simulink model "SingleVehicle_HIL"  (R2016b)
settings: Solver=ode4  StartTime=0.0  StopTime=inf  FixedStep=0.01  RelTol=1e-3  EnableMultiTasking=on
undefined symbols (not defined in the file or in its folder): Angular, dpsi, FromPrescan, IdealSensors, Linear, psi, RHSC, RHSCCmdBus, v, wpFollower, y
undefined symbols (not defined in the file): vd
libraries: robotlib x6, sldrtlib x1
(part 1 of 2)
Description:
  | Real-Time Van der Pol Simulation
  | 
  | The example model "sldrtex_vdp" shows a real-time version of the Simulink(R) Van der Pol
  | simulation model. This model does not need any external signals, so it does
  | not need any data acquisition hardware or driver. This makes the model ideal
  | for the first experiments with Simulink Desktop Real-Time(TM), without need to
  | worry about proper I/O hardware configuration.
  | 
  | How to run this model in Normal Mode:
  | 
  | 1) Double-click the orange button to switch to Normal Mode if needed.
  | 2) Start the real-time execution using Simulation->Run.
  | 3) Observe any missed ticks on the Missed Ticks scope.
  | 
  | How to run this model in External Mode:
  | 
  | 1) Double-click the orange button to switch to External Mode if needed.
  | 2) Start the real-time execution using Simulation->Run. The model will automatically
  |    build, connect to Simulink in External Mode and start.
  | 3) Missed ticks will be always zero.
settings Model: ExtModeTrigDuration=101  Creator=The MathWorks, Inc.  LastModifiedBy=yutongli
settings DataIOCC: LimitDataPoints=on  SignalLoggingName=logsOut
settings OptimizationCC: ExpressionDepthLimit=2147483647  InitFltsAndDblsToZero=on  EfficientMapNaN2IntZero=off  LifeSpan=inf
settings DebuggingCC: UnderspecifiedInitializationDetection=Classic  MergeDetectMultiDrivingBlocksExec=none  SignalResolutionControl=TryResolveAllWithWarning  FcnCallInpInsideContextMsg=warning  AllowSymbolicDim=off  StateNameClashWarn=warning  SFUnexpectedBacktrackingDiag=warning  SFNoUnconditionalDefaultTransitionDiag=warning  SFExecutionAtInitializationDiag=none
settings HardwareCC: TargetBitPerLong=64  TargetBitPerPointer=64  TargetBitPerSizeT=64  TargetBitPerPtrDiffT=64  TargetIntDivRoundTo=Zero  TargetEndianess=LittleEndian  TargetWordSize=64  TargetHWDeviceType=Intel->x86-64
settings ModelReferenceCC: PropagateSignalLabelsOutOfModel=off
settings RTWCC: SystemTargetFile=sldrt.tlc  TemplateMakefile=sldrt.tmf  Description=Simulink Desktop Real-Time  RTWCompilerOptimization=on
settings CodeAppCC: MaxIdLength=95
settings SimulinkDesktopRealTimeCC: TargetPreCompLibLocation=C:\Program Files\MATLAB\R2016B\toolbox\sldrt\lib\win64  TargetLangStandard=C89/C90 (ANSI)  GeneratePreprocessorConditionals=Disable all  SupportVariableSizeSignals=off
settings ConfigComp: CovMetricSettings=dw  CovHtmlReporting=on  CovSaveCumulativeToWorkspaceVar=on  CovSaveSingleToWorkspaceVar=on  CovShowResultsExplorer=off  CovExternalEMLEnable=off  CovSFcnEnable=off

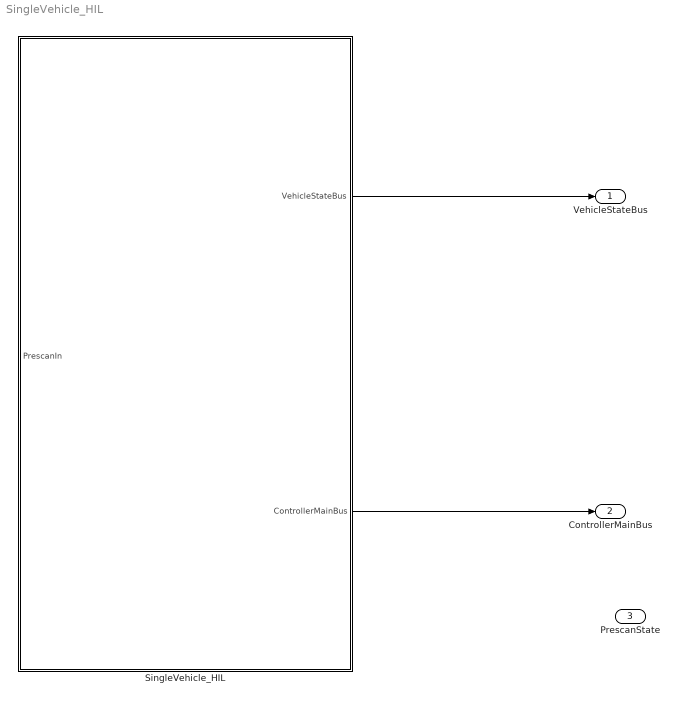
== system SingleVehicle_HIL ==
  SingleVehicle_HIL : Subsystem  mask{veh_struct=vd}
      mask prompts: veh_struct "Vehicle Parameter Structure"
      mask init:
      | set_param([gcb,'/Monitor/VehicleStateBusStorage'],'VariableName',[get_param(gcb,'MaskValueString'),'_DataVehicleBus']);
      | set_param([gcb,'/Monitor/ControllerMainBusStorage/ArbitratedActuationReqStorage'],'VariableName', ...
      |     [get_param(gcb,'MaskValueString'),'_DataControllerMain_ArbitrationActuationReq']);
      | set_param([gcb,'/Monitor/ControllerMainBusStorage/wpFollowerStorage'],'VariableName', ...
      |     [get_param(gcb,'MaskValueString'),'_DataControllerMain_wpFollower']);
      | set_param([gcb,'/Monitor/ControllerMainBusStorage/finalWayPointStorarge'],'VariableName', ...
      |     [get_param(gcb,'MaskValueString'),'_DataControllerMain_finalWayPoint']);
      | set_param([gcb,'/Monitor/ControllerMainBusStorage/currentWayPointStorage'],'VariableName', ...
      |     [get_param(gcb,'MaskValueString'),'_DataControllerMain_currentWayPoint']);
      | set_param([gcb,'/Monitor/ControllerMainBusStorage/wayPointArrayStorage'],'VariableName', ...
      |     [get_param(gcb,'MaskValueString'),'_DataControllerMain_wayPointArray']);
      | set_param([gcb,'/Monitor/ControllerMainBusStorage/selfAwareessBusStorage'],'VariableName', ...
      |     [get_param(gcb,'MaskValueString'),'_DataControllerMain_selfAwareessBus']);
      | set_param([gcb,'/Monitor/ControllerMainBusStorage/IdealSensorsStorage'],'VariableName', ...
      |     [get_param(gcb,'MaskValueString'),'_DataControllerMain_IdealSensors']);
      | set_param([gcb,'/Monitor/ControllerMainBusStorage/FromPrescanStorage'],'VariableName', ...
      |     [get_param(gcb,'MaskValueString'),'_DataControllerMain_FromPrescan']);
  VehicleStateBus : Outport
  ControllerMainBus : Outport  Port=2
  PrescanState : Outport  Port=3
  wires:
  SingleVehicle_HIL/1(VehicleStateBus) -> VehicleStateBus/1
  SingleVehicle_HIL/2(ControllerMainBus) -> ControllerMainBus/1
  ? -> PrescanState/1

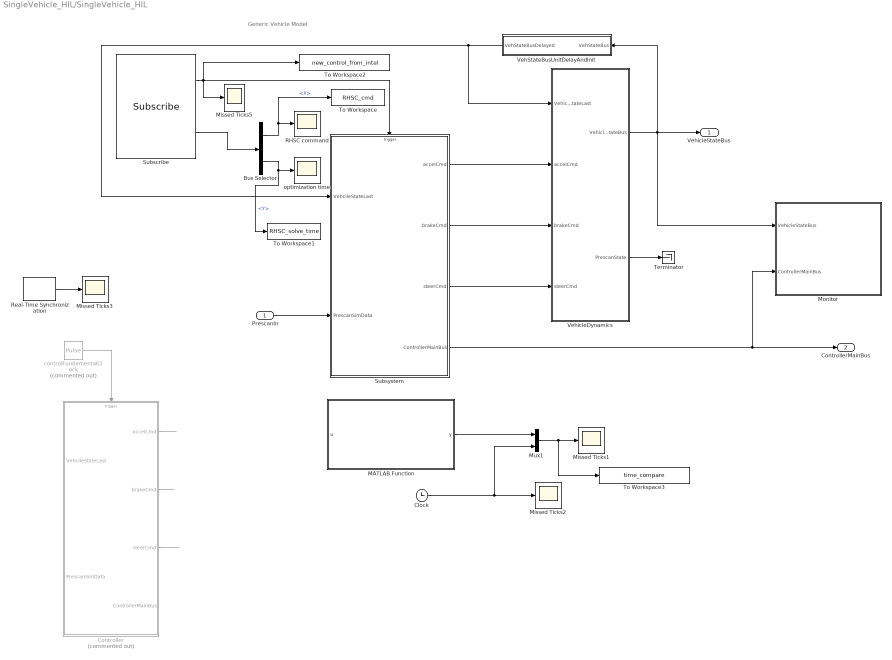
== system SingleVehicle_HIL/SingleVehicle_HIL ==
  note: Generic Vehicle Model
  PrescanIn : Inport
  Bus Selector : BusSelector  OutputSignals=Linear.X,Linear.Y
  Clock : Clock
  Controller : Subsystem  Commented=on
  MATLAB Function : MATLAB Function  TreatAsAtomicUnit=on
  Missed Ticks{1..3,5} (4 alike) : Scope
  Monitor : Subsystem
  Mux1 : Mux  Inputs=2
  RHSC command : Scope
  Real-Time Synchronization : sldrtlib/Real-Time Synchronization  SampleTime=0.01  MaxMissedTicks=1000  ShowMissedTicks=on  YieldWhenWaiting=off
  Subscribe : robotlib/Subscribe  SourceLibraryInfo=This block requires Robotics System Toolbox  topicSource=Select from ROS network  topic=/RHSC_cmd  messageType=geometry_msgs/Twist  sampleTime=-1  messageQueueLength=1
  Subsystem : Subsystem
  Terminator : Terminator
  To Workspace : ToWorkspace  VariableName=RHSC_cmd  SaveFormat=Structure With Time  SampleTime=-1
  To Workspace1 : ToWorkspace  VariableName=RHSC_solve_time  SaveFormat=Structure With Time  SampleTime=-1
  To Workspace2 : ToWorkspace  VariableName=new_control_from_intel  SaveFormat=Structure With Time  SampleTime=-1
  To Workspace3 : ToWorkspace  VariableName=time_compare  SaveFormat=Structure With Time  SampleTime=-1
  VehStateBusUnitDelayAndInit : Subsystem
  VehicleDynamics : Subsystem
  controlFundamentalClock : DiscretePulseGenerator  Commented=on  PulseType=Time based  Period=veh_struct.CONTROL_OS_SAMPLETIME  PulseWidth=5
  optimization time : Scope
  VehicleStateBus : Outport
  ControllerMainBus : Outport  Port=2
  wires:
  PrescanIn/1 -> Subsystem/2(PrescanSimData)
  Controller/1(accelCmd) -> ?
  Controller/2(brakeCmd) -> ?
  Controller/3(steerCmd) -> ?
  VehicleDynamics/1(VehicleStateBus) -> VehStateBusUnitDelayAndInit/1(VehStateBus), Monitor/1(VehicleStateBus), VehicleStateBus/1
  VehStateBusUnitDelayAndInit/1(VehStateBusDelayed) -> Subsystem/1(VehcileStateLast), VehicleDynamics/1(VehicleStateLast)
  controlFundamentalClock/1 -> Controller/Trigger
  Real-Time Synchronization/1 -> Missed Ticks3/1
  MATLAB Function/1(y) -> Mux1/1
  Mux1/1 -> To Workspace3/1, Missed Ticks1/1
  Clock/1 -> Missed Ticks2/1, Mux1/2
  Subscribe/1 -> To Workspace2/1, Subsystem/Trigger, Missed Ticks5/1
  Subscribe/2 -> Bus Selector/1
  Bus Selector/1 -> RHSC command/1, To Workspace/1  "<X>"
  Subsystem/4(ControllerMainBus) -> Monitor/2(ControllerMainBus), ControllerMainBus/1
  Subsystem/1(accelCmd) -> VehicleDynamics/2(accelCmd)
  Subsystem/2(brakeCmd) -> VehicleDynamics/3(brakeCmd)
  Subsystem/3(steerCmd) -> VehicleDynamics/4(steerCmd)
  VehicleDynamics/2(PrescanState) -> Terminator/1
  Bus Selector/2 -> To Workspace1/1, optimization time/1  "<Y>"

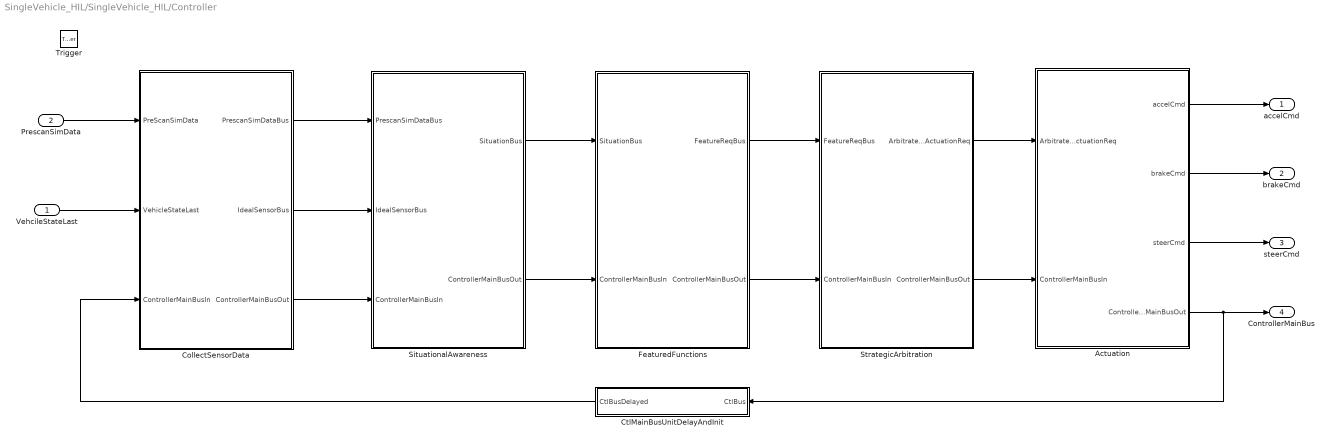
== system SingleVehicle_HIL/SingleVehicle_HIL/Controller ==
  VehcileStateLast : Inport
  PrescanSimData : Inport  Port=2
  Trigger : TriggerPort  VariantControl=Variant  PortDimensions=1
  Actuation : Subsystem
  CollectSensorData : Subsystem
  CtlMainBusUnitDelayAndInit : Subsystem
  FeaturedFunctions : Subsystem
  SituationalAwareness : Subsystem
  StrategicArbitration : Subsystem
  accelCmd : Outport
  brakeCmd : Outport  Port=2
  steerCmd : Outport  Port=3
  ControllerMainBus : Outport  Port=4
  wires:
  PrescanSimData/1 -> CollectSensorData/1(PreScanSimData)
  Actuation/1(accelCmd) -> accelCmd/1
  Actuation/2(brakeCmd) -> brakeCmd/1
  Actuation/3(steerCmd) -> steerCmd/1
  StrategicArbitration/1(ArbitratedActuationReq) -> Actuation/1(ArbitratedActuationReq)
  StrategicArbitration/2(ControllerMainBusOut) -> Actuation/2(ControllerMainBusIn)
  FeaturedFunctions/2(ControllerMainBusOut) -> StrategicArbitration/2(ControllerMainBusIn)
  FeaturedFunctions/1(FeatureReqBus) -> StrategicArbitration/1(FeatureReqBus)
  SituationalAwareness/1(SituationBus) -> FeaturedFunctions/1(SituationBus)
  SituationalAwareness/2(ControllerMainBusOut) -> FeaturedFunctions/2(ControllerMainBusIn)
  CollectSensorData/3(ControllerMainBusOut) -> SituationalAwareness/3(ControllerMainBusIn)
  VehcileStateLast/1 -> CollectSensorData/2(VehicleStateLast)
  Actuation/4(ControllerMainBusOut) -> CtlMainBusUnitDelayAndInit/1(CtlBus), ControllerMainBus/1
  CtlMainBusUnitDelayAndInit/1(CtlBusDelayed) -> CollectSensorData/3(ControllerMainBusIn)
  CollectSensorData/1(PrescanSimDataBus) -> SituationalAwareness/1(PrescanSimDataBus)
  CollectSensorData/2(IdealSensorBus) -> SituationalAwareness/2(IdealSensorBus)

== system SingleVehicle_HIL/SingleVehicle_HIL/Monitor ==
  VehicleStateBus : Inport
  ControllerMainBus : Inport  Port=2
  ControllerMainBusStorage : Subsystem
  VehicleStateBusStorage : ToWorkspace  VariableName=vd_DataVehicleBus  SaveFormat=Timeseries  SampleTime=-1
  wires:
  VehicleStateBus/1 -> VehicleStateBusStorage/1
  ControllerMainBus/1 -> ControllerMainBusStorage/1(ControllerMainBus)

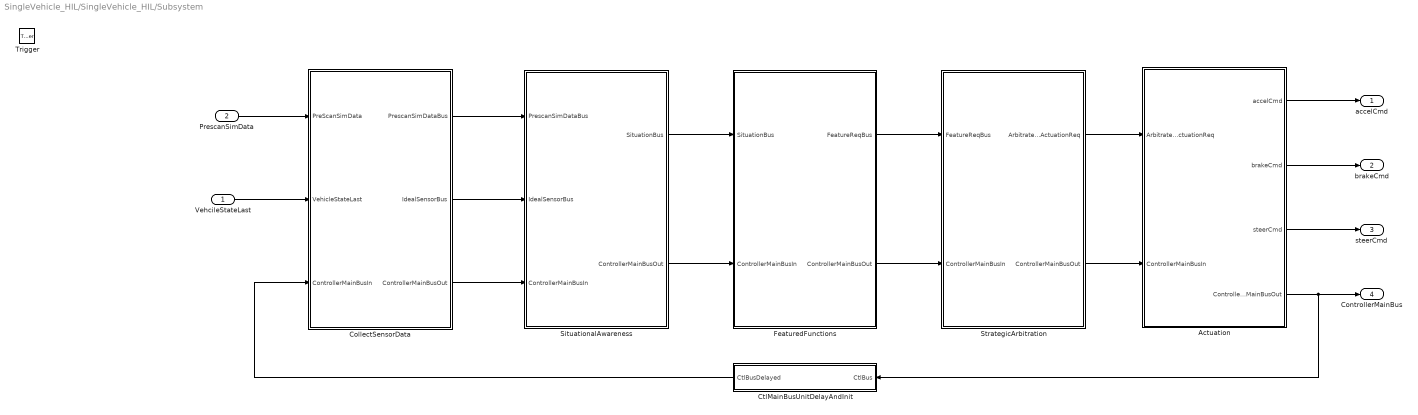
== system SingleVehicle_HIL/SingleVehicle_HIL/Subsystem ==
  VehcileStateLast : Inport
  PrescanSimData : Inport  Port=2
  Trigger : TriggerPort  VariantControl=Variant  PortDimensions=1
  Actuation : Subsystem
  CollectSensorData : Subsystem
  CtlMainBusUnitDelayAndInit : Subsystem
  FeaturedFunctions : Subsystem
  SituationalAwareness : Subsystem
  StrategicArbitration : Subsystem
  accelCmd : Outport
  brakeCmd : Outport  Port=2
  steerCmd : Outport  Port=3
  ControllerMainBus : Outport  Port=4
  wires:
  PrescanSimData/1 -> CollectSensorData/1(PreScanSimData)
  Actuation/1(accelCmd) -> accelCmd/1
  Actuation/2(brakeCmd) -> brakeCmd/1
  Actuation/3(steerCmd) -> steerCmd/1
  StrategicArbitration/1(ArbitratedActuationReq) -> Actuation/1(ArbitratedActuationReq)
  StrategicArbitration/2(ControllerMainBusOut) -> Actuation/2(ControllerMainBusIn)
  FeaturedFunctions/2(ControllerMainBusOut) -> StrategicArbitration/2(ControllerMainBusIn)
  FeaturedFunctions/1(FeatureReqBus) -> StrategicArbitration/1(FeatureReqBus)
  SituationalAwareness/1(SituationBus) -> FeaturedFunctions/1(SituationBus)
  SituationalAwareness/2(ControllerMainBusOut) -> FeaturedFunctions/2(ControllerMainBusIn)
  CollectSensorData/3(ControllerMainBusOut) -> SituationalAwareness/3(ControllerMainBusIn)
  VehcileStateLast/1 -> CollectSensorData/2(VehicleStateLast)
  Actuation/4(ControllerMainBusOut) -> CtlMainBusUnitDelayAndInit/1(CtlBus), ControllerMainBus/1
  CtlMainBusUnitDelayAndInit/1(CtlBusDelayed) -> CollectSensorData/3(ControllerMainBusIn)
  CollectSensorData/1(PrescanSimDataBus) -> SituationalAwareness/1(PrescanSimDataBus)
  CollectSensorData/2(IdealSensorBus) -> SituationalAwareness/2(IdealSensorBus)

== system SingleVehicle_HIL/SingleVehicle_HIL/VehStateBusUnitDelayAndInit ==
  VehStateBus : Inport
  MATLAB Function : MATLAB Function  TreatAsAtomicUnit=on
  Memory : Memory  InheritSampleTime=on
  VehStateBusDelayed : Outport
  wires:
  Memory/1 -> MATLAB Function/1(u)
  VehStateBus/1 -> Memory/1
  MATLAB Function/1(y) -> VehStateBusDelayed/1

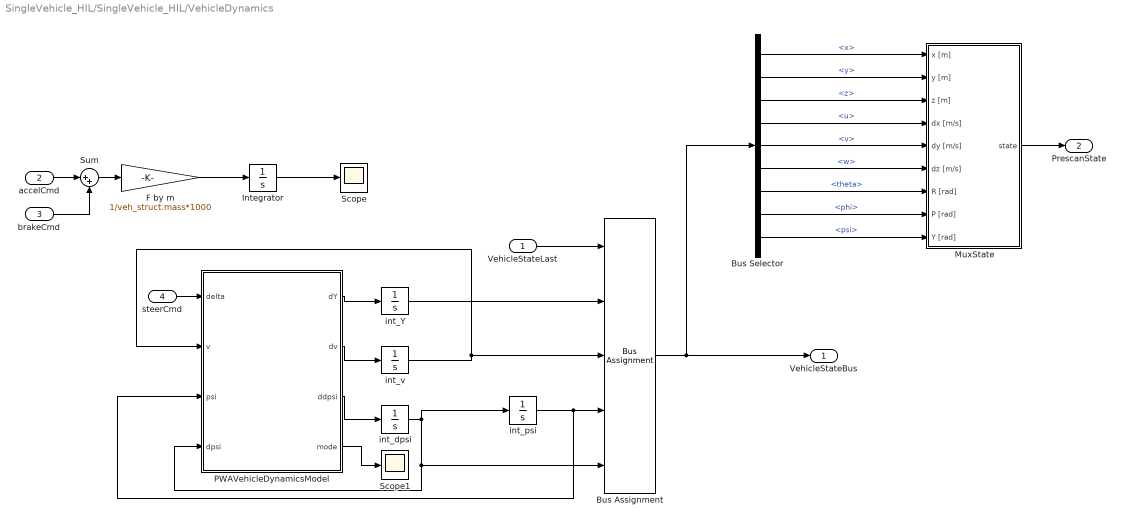
== system SingleVehicle_HIL/SingleVehicle_HIL/VehicleDynamics ==
  VehicleStateLast : Inport
  accelCmd : Inport  Port=2
  brakeCmd : Inport  Port=3
  steerCmd : Inport  Port=4
  Bus Assignment : BusAssignment  AssignedSignals=y,v,psi,dpsi
  Bus Selector : BusSelector  OutputSignals=x,y,z,u,v,w,theta,phi,psi
  F by m : Gain  Gain=1/veh_struct.mass*1000
  Integrator : Integrator  InitialCondition=veh_struct.init.u
  MuxState : Subsystem  Tag=MuxState  mask(Empty Dynamics State Block){positioningmode=on, TimeStep=1/20}
      mask prompts: positioningmode "Positioning Mode"; TimeStep "Auto Assigned: Time Step [s]"
      mask help:
      | Build the state of an actor based on user input.
      | The user can either use positioning mode or dynamics mode.
      | - When using positioning mode the position and orientation of the actor are set directly based on the input. Expected input is relative to the initial position and orientation of the actor. It's also possible to specify the velocity of the actor, though this input isn't used, only passed on.
      | - When using dynamics mode the position input is ignored. Expected input is velocity and orientation. The velocity is relative the current orientation of the actor, while orientation is relative to its initial orientation. The position of the actor is calculated based on the velocity and orientation given.
      settings: DeleteFcn=PreScanBlockDeleteFcn;
  PWAVehicleDynamicsModel : MATLAB Function  TreatAsAtomicUnit=on
  Scope : Scope
  Scope1 : Scope
  Sum : Sum  Inputs=|++
  int_Y : Integrator  InitialCondition=veh_struct.init.Y
  int_dpsi : Integrator  InitialCondition=veh_struct.init.dpsi
  int_psi : Integrator  InitialCondition=veh_struct.init.psi
  int_v : Integrator  InitialCondition=veh_struct.init.v
  VehicleStateBus : Outport
  PrescanState : Outport  Port=2
  wires:
  MuxState/1(state) -> PrescanState/1
  Bus Assignment/1 -> VehicleStateBus/1, Bus Selector/1
  Bus Selector/3 -> MuxState/3(z [m])  "<z>"
  Bus Selector/4 -> MuxState/4(dx [m/s])  "<u>"
  Bus Selector/5 -> MuxState/5(dy [m/s])  "<v>"
  Bus Selector/6 -> MuxState/6(dz [m/s])  "<w>"
  Bus Selector/1 -> MuxState/1(x [m])  "<x>"
  Bus Selector/2 -> MuxState/2(y [m])  "<y>"
  Bus Selector/7 -> MuxState/7(R [rad])  "<theta>"
  Bus Selector/9 -> MuxState/9(Y [rad])  "<psi>"
  Bus Selector/8 -> MuxState/8(P [rad])  "<phi>"
  VehicleStateLast/1 -> Bus Assignment/1
  accelCmd/1 -> Sum/1
  brakeCmd/1 -> Sum/2
  Sum/1 -> F by m/1
  F by m/1 -> Integrator/1
  Integrator/1 -> Scope/1
  steerCmd/1 -> PWAVehicleDynamicsModel/1(delta)
  PWAVehicleDynamicsModel/2(dv) -> int_v/1
  int_v/1 -> PWAVehicleDynamicsModel/2(v), Bus Assignment/3
  PWAVehicleDynamicsModel/3(ddpsi) -> int_dpsi/1
  int_dpsi/1 -> int_psi/1, PWAVehicleDynamicsModel/4(dpsi), Bus Assignment/5
  PWAVehicleDynamicsModel/1(dY) -> int_Y/1
  int_Y/1 -> Bus Assignment/2
  int_psi/1 -> PWAVehicleDynamicsModel/3(psi), Bus Assignment/4
  PWAVehicleDynamicsModel/4(mode) -> Scope1/1

== system SingleVehicle_HIL/SingleVehicle_HIL/Controller/Actuation ==
  ArbitratedActuationReq : Inport
  ControllerMainBusIn : Inport  Port=2
  ActuatorDrivers : Subsystem  TreatAsAtomicUnit=on
  Bus Assignment : BusAssignment  AssignedSignals=ActuationCmdBus
  Bus Selector : BusSelector  OutputSignals=ActuationCmdBus
  DynamicControls : Subsystem  TreatAsAtomicUnit=on
  accelCmd : Outport
  brakeCmd : Outport  Port=2
  steerCmd : Outport  Port=3
  ControllerMainBusOut : Outport  Port=4
  wires:
  ControllerMainBusIn/1 -> DynamicControls/2(Ctl), Bus Assignment/1, Bus Selector/1
  ArbitratedActuationReq/1 -> DynamicControls/1(ActReq)
  Bus Selector/1 -> DynamicControls/3(ActCmdsPrev)  "<ActuationCmdBus>"
  DynamicControls/1(ActCmds) -> ActuatorDrivers/1(ActCmds), Bus Assignment/2
  Bus Assignment/1 -> ControllerMainBusOut/1
  ActuatorDrivers/2(decel_cmd) -> brakeCmd/1
  ActuatorDrivers/1(accel_cmd) -> accelCmd/1
  ActuatorDrivers/3(steering_cmd) -> steerCmd/1

== system SingleVehicle_HIL/SingleVehicle_HIL/Controller/CollectSensorData ==
  PreScanSimData : Inport
  VehicleStateLast : Inport  Port=2
  ControllerMainBusIn : Inport  Port=3
  Bus Assignment : BusAssignment  AssignedSignals=FromPrescan,IdealSensors
  IdealSensorsProcess : Subsystem
  PrescanProcess : Subsystem
  PrescanSimDataBus : Outport
  IdealSensorBus : Outport  Port=2
  ControllerMainBusOut : Outport  Port=3
  wires:
  PreScanSimData/1 -> PrescanProcess/1(PrescanSimData)
  PrescanProcess/1(PrescanSimDataBus) -> Bus Assignment/2, PrescanSimDataBus/1
  VehicleStateLast/1 -> IdealSensorsProcess/1(VehicleState)
  IdealSensorsProcess/1(IdealSensorsBus) -> IdealSensorBus/1, Bus Assignment/3
  Bus Assignment/1 -> ControllerMainBusOut/1
  ControllerMainBusIn/1 -> Bus Assignment/1

== system SingleVehicle_HIL/SingleVehicle_HIL/Controller/CtlMainBusUnitDelayAndInit ==
  CtlBus : Inport
  MATLAB Function : Subsystem  TreatAsAtomicUnit=on
  Memory : Memory  InheritSampleTime=on
  CtlBusDelayed : Outport
  wires:
  Memory/1 -> MATLAB Function/1(u)
  CtlBus/1 -> Memory/1
  MATLAB Function/1(y) -> CtlBusDelayed/1

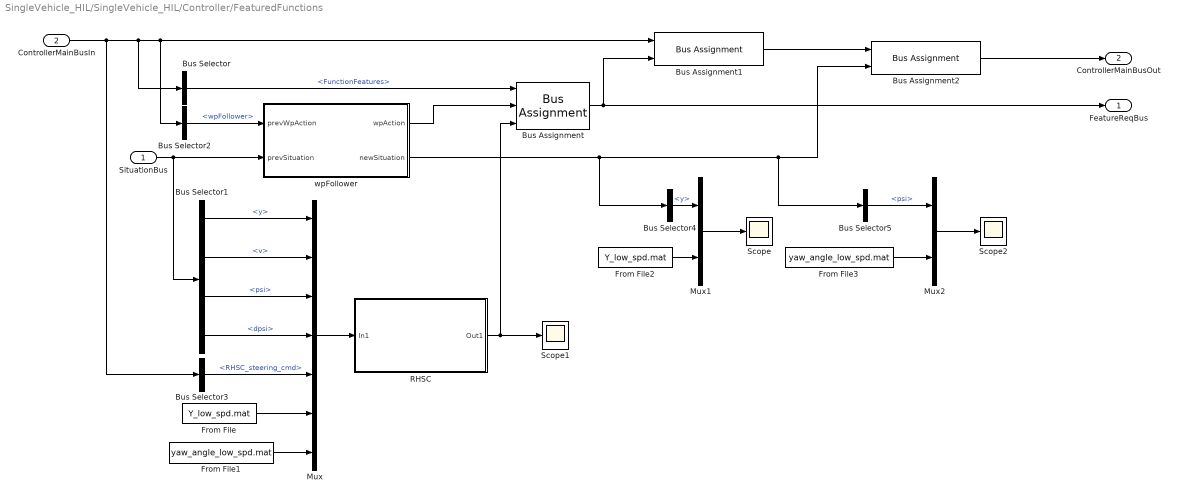
== system SingleVehicle_HIL/SingleVehicle_HIL/Controller/FeaturedFunctions ==
  SituationBus : Inport
  ControllerMainBusIn : Inport  Port=2
  Bus Assignment : BusAssignment  AssignedSignals=wpFollower,RHSCCmdBus.RHSC_steering_cmd
  Bus Assignment1 : BusAssignment  AssignedSignals=FunctionFeatures
  Bus Assignment2 : BusAssignment  AssignedSignals=situationBus
  Bus Selector : BusSelector  OutputSignals=FunctionFeatures
  Bus Selector1 : BusSelector  OutputSignals=selfAwarenessBus.y,selfAwarenessBus.v,selfAwarenessBus.psi,selfAwarenessBus.dpsi
  Bus Selector2 : BusSelector  OutputSignals=FunctionFeatures.wpFollower
  Bus Selector3 : BusSelector  OutputSignals=FunctionFeatures.RHSCCmdBus.RHSC_steering_cmd
  Bus Selector4 : BusSelector  OutputSignals=selfAwarenessBus.y
  Bus Selector5 : BusSelector  OutputSignals=selfAwarenessBus.psi
  From File : FromFile  FileName=Y_low_spd.mat
  From File1 : FromFile  FileName=yaw_angle_low_spd.mat
  From File2 : FromFile  FileName=Y_low_spd.mat
  From File3 : FromFile  FileName=yaw_angle_low_spd.mat
  Mux : Mux  Inputs=7
  Mux1 : Mux  Inputs=2
  Mux2 : Mux  Inputs=2
  RHSC : Subsystem
  Scope : Scope
  Scope1 : Scope
  Scope2 : Scope
  wpFollower : Subsystem  TreatAsAtomicUnit=on
  FeatureReqBus : Outport
  ControllerMainBusOut : Outport  Port=2
  wires:
  ControllerMainBusIn/1 -> Bus Selector3/1, Bus Selector/1, Bus Selector2/1, Bus Assignment1/1
  Bus Selector/1 -> Bus Assignment/1  "<FunctionFeatures>"
  wpFollower/1(wpAction) -> Bus Assignment/2
  Bus Assignment/1 -> Bus Assignment1/2, FeatureReqBus/1
  Bus Assignment1/1 -> Bus Assignment2/1
  wpFollower/2(newSituation) -> Bus Selector4/1, Bus Selector5/1, Bus Assignment2/2
  Bus Assignment2/1 -> ControllerMainBusOut/1
  Bus Selector2/1 -> wpFollower/1(prevWpAction)  "<wpFollower>"
  SituationBus/1 -> Bus Selector1/1, wpFollower/2(prevSituation)
  Bus Selector3/1 -> Mux/5  "<RHSC_steering_cmd>"
  RHSC/1(Out1) -> Scope1/1, Bus Assignment/3
  Mux/1 -> RHSC/1(In1)
  Bus Selector1/1 -> Mux/1  "<y>"
  Bus Selector1/2 -> Mux/2  "<v>"
  Bus Selector1/3 -> Mux/3  "<psi>"
  Bus Selector1/4 -> Mux/4  "<dpsi>"
  From File/1 -> Mux/6
  From File1/1 -> Mux/7
  Bus Selector4/1 -> Mux1/1  "<y>"
  From File2/1 -> Mux1/2
  Mux1/1 -> Scope/1
  Bus Selector5/1 -> Mux2/1  "<psi>"
  From File3/1 -> Mux2/2
  Mux2/1 -> Scope2/1

== system SingleVehicle_HIL/SingleVehicle_HIL/Controller/SituationalAwareness ==
  PrescanSimDataBus : Inport
  IdealSensorBus : Inport  Port=2
  ControllerMainBusIn : Inport  Port=3
  Bus Assignment : BusAssignment  AssignedSignals=situationBus
  Bus Selector : BusSelector  OutputSignals=situationBus
  situationAwareness : Subsystem  TreatAsAtomicUnit=on
  SituationBus : Outport
  ControllerMainBusOut : Outport  Port=2
  wires:
  ControllerMainBusIn/1 -> Bus Assignment/1, Bus Selector/1
  Bus Selector/1 -> situationAwareness/1(prevSituation)  "<situationBus>"
  PrescanSimDataBus/1 -> situationAwareness/2(prescanSimData)
  IdealSensorBus/1 -> situationAwareness/3(idealSensors)
  situationAwareness/1(newSituation) -> Bus Assignment/2, SituationBus/1
  Bus Assignment/1 -> ControllerMainBusOut/1

== system SingleVehicle_HIL/SingleVehicle_HIL/Controller/StrategicArbitration ==
  FeatureReqBus : Inport
  ControllerMainBusIn : Inport  Port=2
  Arbitration : Subsystem  TreatAsAtomicUnit=on
  Bus Assignment : BusAssignment  AssignedSignals=ArbitratedActuationReq
  ArbitratedActuationReq : Outport
  ControllerMainBusOut : Outport  Port=2
  wires:
  FeatureReqBus/1 -> Arbitration/1(FunctionFeatures)
  Arbitration/1(ArbitratedReq) -> Bus Assignment/2, ArbitratedActuationReq/1
  ControllerMainBusIn/1 -> Bus Assignment/1
  Bus Assignment/1 -> ControllerMainBusOut/1

== system SingleVehicle_HIL/SingleVehicle_HIL/Monitor/ControllerMainBusStorage ==
  ControllerMainBus : Inport
  ArbitratedActuationReqStorage : ToWorkspace  VariableName=vd_DataControllerMain_ArbitrationActuationReq  SaveFormat=Timeseries  SampleTime=-1
  Bus Selector : BusSelector  OutputSignals=ArbitratedActuationReq,FunctionFeatures.wpFollower,situationBus.wP.finalWayPoint,situationBus.wP.currentWayPoint,situationBus.wP.wayPointArray,situationBus.selfAwarenessBus,IdealSensors,FromPrescan
  FromPrescanStorage : ToWorkspace  VariableName=vd_DataControllerMain_FromPrescan  SaveFormat=Timeseries  SampleTime=-1
  IdealSensorsStorage : ToWorkspace  VariableName=vd_DataControllerMain_IdealSensors  SaveFormat=Timeseries  SampleTime=-1
  currentWayPointStorage : ToWorkspace  VariableName=vd_DataControllerMain_currentWayPoint  SaveFormat=Timeseries  SampleTime=-1
  finalWayPointStorarge : ToWorkspace  VariableName=vd_DataControllerMain_finalWayPoint  SaveFormat=Timeseries  SampleTime=-1
  selfAwareessBusStorage : ToWorkspace  VariableName=vd_DataControllerMain_selfAwareessBus  SaveFormat=Timeseries  SampleTime=-1
  wayPointArrayStorage : ToWorkspace  VariableName=vd_DataControllerMain_wayPointArray  SampleTime=-1
  wpFollowerStorage : ToWorkspace  VariableName=vd_DataControllerMain_wpFollower  SaveFormat=Timeseries  SampleTime=-1
  wires:
  ControllerMainBus/1 -> Bus Selector/1
  Bus Selector/1 -> ArbitratedActuationReqStorage/1  "<ArbitratedActuationReq>"
  Bus Selector/2 -> wpFollowerStorage/1  "<wpFollower>"
  Bus Selector/3 -> finalWayPointStorarge/1  "<finalWayPoint>"
  Bus Selector/8 -> FromPrescanStorage/1  "<FromPrescan>"
  Bus Selector/6 -> selfAwareessBusStorage/1  "<selfAwarenessBus>"
  Bus Selector/4 -> currentWayPointStorage/1  "<currentWayPoint>"
  Bus Selector/7 -> IdealSensorsStorage/1  "<IdealSensors>"

== system SingleVehicle_HIL/SingleVehicle_HIL/Subsystem/Actuation ==
  ArbitratedActuationReq : Inport
  ControllerMainBusIn : Inport  Port=2
  ActuatorDrivers : MATLAB Function  TreatAsAtomicUnit=on
  Bus Assignment : BusAssignment  AssignedSignals=ActuationCmdBus
  Bus Selector : BusSelector  OutputSignals=ActuationCmdBus
  DynamicControls : MATLAB Function  TreatAsAtomicUnit=on
  accelCmd : Outport
  brakeCmd : Outport  Port=2
  steerCmd : Outport  Port=3
  ControllerMainBusOut : Outport  Port=4
  wires:
  ControllerMainBusIn/1 -> DynamicControls/2(Ctl), Bus Assignment/1, Bus Selector/1
  ArbitratedActuationReq/1 -> DynamicControls/1(ActReq)
  Bus Selector/1 -> DynamicControls/3(ActCmdsPrev)  "<ActuationCmdBus>"
  DynamicControls/1(ActCmds) -> ActuatorDrivers/1(ActCmds), Bus Assignment/2
  Bus Assignment/1 -> ControllerMainBusOut/1
  ActuatorDrivers/2(decel_cmd) -> brakeCmd/1
  ActuatorDrivers/1(accel_cmd) -> accelCmd/1
  ActuatorDrivers/3(steering_cmd) -> steerCmd/1

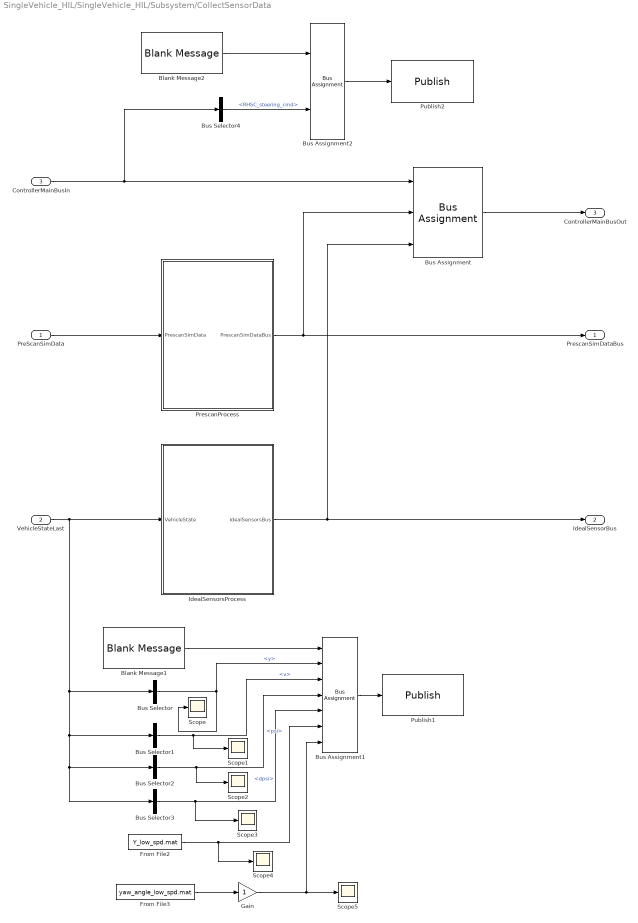
== system SingleVehicle_HIL/SingleVehicle_HIL/Subsystem/CollectSensorData ==
  PreScanSimData : Inport
  VehicleStateLast : Inport  Port=2
  ControllerMainBusIn : Inport  Port=3
  Blank Message1 : robotlib/Blank Message  SourceLibraryInfo=This block requires Robotics System Toolbox  messageType=geometry_msgs/Twist  SampleTime=-1
  Blank Message2 : robotlib/Blank Message  SourceLibraryInfo=This block requires Robotics System Toolbox  messageType=geometry_msgs/Twist  SampleTime=-1
  Bus Assignment : BusAssignment  AssignedSignals=FromPrescan,IdealSensors
  Bus Assignment1 : BusAssignment  AssignedSignals=Linear.X,Linear.Y,Angular.Z,Angular.Y,Linear.Z,Angular.X
  Bus Assignment2 : BusAssignment  AssignedSignals=Linear.X
  Bus Selector : BusSelector  OutputSignals=y
  Bus Selector1 : BusSelector  OutputSignals=v
  Bus Selector2 : BusSelector  OutputSignals=psi
  Bus Selector3 : BusSelector  OutputSignals=dpsi
  Bus Selector4 : BusSelector  OutputSignals=FunctionFeatures.RHSCCmdBus.RHSC_steering_cmd
  From File2 : FromFile  FileName=Y_low_spd.mat
  From File3 : FromFile  FileName=yaw_angle_low_spd.mat
  Gain : Gain
  IdealSensorsProcess : Subsystem
  PrescanProcess : Subsystem
  Publish1 : robotlib/Publish  SourceLibraryInfo=This block requires Robotics System Toolbox  topicSource=Specify your own  topic=/veh_state  messageType=geometry_msgs/Twist  messageQueueLength=10
  Publish2 : robotlib/Publish  SourceLibraryInfo=This block requires Robotics System Toolbox  topicSource=Specify your own  topic=/old_u  messageType=geometry_msgs/Twist  messageQueueLength=10
  Scope{,1..5} (6 alike) : Scope
  PrescanSimDataBus : Outport
  IdealSensorBus : Outport  Port=2
  ControllerMainBusOut : Outport  Port=3
  wires:
  PreScanSimData/1 -> PrescanProcess/1(PrescanSimData)
  PrescanProcess/1(PrescanSimDataBus) -> Bus Assignment/2, PrescanSimDataBus/1
  VehicleStateLast/1 -> Bus Selector3/1, Bus Selector2/1, Bus Selector1/1, Bus Selector/1, IdealSensorsProcess/1(VehicleState)
  IdealSensorsProcess/1(IdealSensorsBus) -> IdealSensorBus/1, Bus Assignment/3
  Bus Assignment/1 -> ControllerMainBusOut/1
  ControllerMainBusIn/1 -> Bus Selector4/1, Bus Assignment/1
  Bus Selector2/1 -> Scope2/1, Bus Assignment1/4  "<psi>"
  Bus Selector1/1 -> Scope1/1, Bus Assignment1/3  "<v>"
  Blank Message1/1 -> Bus Assignment1/1
  Bus Assignment1/1 -> Publish1/1
  Bus Selector/1 -> Bus Assignment1/2, Scope/1  "<y>"
  Bus Selector3/1 -> Scope3/1, Bus Assignment1/5  "<dpsi>"
  From File2/1 -> Scope4/1, Bus Assignment1/6
  From File3/1 -> Gain/1
  Blank Message2/1 -> Bus Assignment2/1
  Bus Selector4/1 -> Bus Assignment2/2  "<RHSC_steering_cmd>"
  Bus Assignment2/1 -> Publish2/1
  Gain/1 -> Scope5/1, Bus Assignment1/7

== system SingleVehicle_HIL/SingleVehicle_HIL/Subsystem/CtlMainBusUnitDelayAndInit ==
  CtlBus : Inport
  MATLAB Function : MATLAB Function  TreatAsAtomicUnit=on
  Memory : Memory  InheritSampleTime=on
  CtlBusDelayed : Outport
  wires:
  Memory/1 -> MATLAB Function/1(u)
  CtlBus/1 -> Memory/1
  MATLAB Function/1(y) -> CtlBusDelayed/1

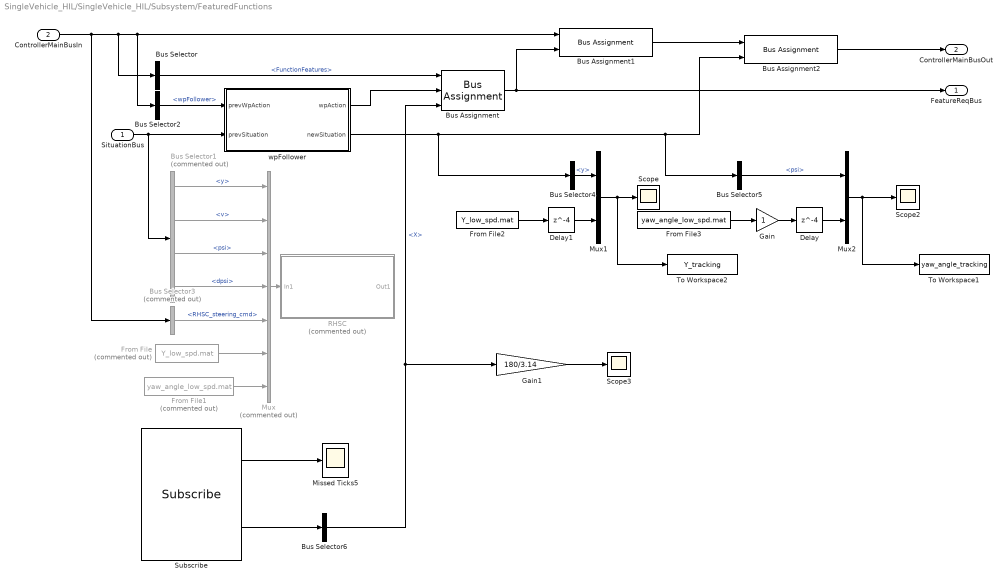
== system SingleVehicle_HIL/SingleVehicle_HIL/Subsystem/FeaturedFunctions ==
  SituationBus : Inport
  ControllerMainBusIn : Inport  Port=2
  Bus Assignment : BusAssignment  AssignedSignals=wpFollower,RHSCCmdBus.RHSC_steering_cmd
  Bus Assignment1 : BusAssignment  AssignedSignals=FunctionFeatures
  Bus Assignment2 : BusAssignment  AssignedSignals=situationBus
  Bus Selector : BusSelector  OutputSignals=FunctionFeatures
  Bus Selector1 : BusSelector  Commented=on  OutputSignals=selfAwarenessBus.y,selfAwarenessBus.v,selfAwarenessBus.psi,selfAwarenessBus.dpsi
  Bus Selector2 : BusSelector  OutputSignals=FunctionFeatures.wpFollower
  Bus Selector3 : BusSelector  Commented=on  OutputSignals=FunctionFeatures.RHSCCmdBus.RHSC_steering_cmd
  Bus Selector4 : BusSelector  OutputSignals=selfAwarenessBus.y
  Bus Selector5 : BusSelector  OutputSignals=selfAwarenessBus.psi
  Bus Selector6 : BusSelector  OutputSignals=Linear.X
  Delay : Delay  DelayLength=4
  Delay1 : Delay  DelayLength=4
  From File : FromFile  Commented=on  FileName=Y_low_spd.mat
  From File1 : FromFile  Commented=on  FileName=yaw_angle_low_spd.mat
  From File2 : FromFile  FileName=Y_low_spd.mat
  From File3 : FromFile  FileName=yaw_angle_low_spd.mat
  Gain : Gain
  Gain1 : Gain  Gain=180/3.14
  Missed Ticks5 : Scope
  Mux : Mux  Commented=on  Inputs=7
  Mux1 : Mux  Inputs=2
  Mux2 : Mux  Inputs=2
  RHSC : Subsystem  Commented=on
  Scope : Scope
  Scope2 : Scope
  Scope3 : Scope
  Subscribe : robotlib/Subscribe  SourceLibraryInfo=This block requires Robotics System Toolbox  topicSource=Select from ROS network  topic=/RHSC_cmd  messageType=geometry_msgs/Twist  sampleTime=-1  messageQueueLength=1
  To Workspace1 : ToWorkspace  VariableName=yaw_angle_tracking  SaveFormat=Structure With Time  SampleTime=-1
  To Workspace2 : ToWorkspace  VariableName=Y_tracking  SaveFormat=Structure With Time  SampleTime=-1
  wpFollower : MATLAB Function  TreatAsAtomicUnit=on
  FeatureReqBus : Outport
  ControllerMainBusOut : Outport  Port=2
  wires:
  ControllerMainBusIn/1 -> Bus Selector3/1, Bus Selector/1, Bus Selector2/1, Bus Assignment1/1
  Bus Selector/1 -> Bus Assignment/1  "<FunctionFeatures>"
  wpFollower/1(wpAction) -> Bus Assignment/2
  Bus Assignment/1 -> Bus Assignment1/2, FeatureReqBus/1
  Bus Assignment1/1 -> Bus Assignment2/1
  wpFollower/2(newSituation) -> Bus Selector5/1, Bus Assignment2/2, Bus Selector4/1
  Bus Assignment2/1 -> ControllerMainBusOut/1
  Bus Selector2/1 -> wpFollower/1(prevWpAction)  "<wpFollower>"
  SituationBus/1 -> Bus Selector1/1, wpFollower/2(prevSituation)
  Bus Selector3/1 -> Mux/5  "<RHSC_steering_cmd>"
  Mux/1 -> RHSC/1(In1)
  Bus Selector1/1 -> Mux/1  "<y>"
  Bus Selector1/2 -> Mux/2  "<v>"
  Bus Selector1/3 -> Mux/3  "<psi>"
  Bus Selector1/4 -> Mux/4  "<dpsi>"
  From File/1 -> Mux/6
  From File1/1 -> Mux/7
  Bus Selector4/1 -> Mux1/1  "<y>"
  From File2/1 -> Delay1/1
  Mux1/1 -> To Workspace2/1, Scope/1
  Bus Selector5/1 -> Mux2/1  "<psi>"
  From File3/1 -> Gain/1
  Mux2/1 -> To Workspace1/1, Scope2/1
  Subscribe/1 -> Missed Ticks5/1
  Subscribe/2 -> Bus Selector6/1
  Bus Selector6/1 -> Gain1/1, Bus Assignment/3  "<X>"
  Gain/1 -> Delay/1
  Gain1/1 -> Scope3/1
  Delay/1 -> Mux2/2
  Delay1/1 -> Mux1/2

== system SingleVehicle_HIL/SingleVehicle_HIL/Subsystem/SituationalAwareness ==
  PrescanSimDataBus : Inport
  IdealSensorBus : Inport  Port=2
  ControllerMainBusIn : Inport  Port=3
  Bus Assignment : BusAssignment  AssignedSignals=situationBus
  Bus Selector : BusSelector  OutputSignals=situationBus
  situationAwareness : MATLAB Function  TreatAsAtomicUnit=on
  SituationBus : Outport
  ControllerMainBusOut : Outport  Port=2
  wires:
  ControllerMainBusIn/1 -> Bus Assignment/1, Bus Selector/1
  Bus Selector/1 -> situationAwareness/1(prevSituation)  "<situationBus>"
  PrescanSimDataBus/1 -> situationAwareness/2(prescanSimData)
  IdealSensorBus/1 -> situationAwareness/3(idealSensors)
  situationAwareness/1(newSituation) -> Bus Assignment/2, SituationBus/1
  Bus Assignment/1 -> ControllerMainBusOut/1

== system SingleVehicle_HIL/SingleVehicle_HIL/Subsystem/StrategicArbitration ==
  FeatureReqBus : Inport
  ControllerMainBusIn : Inport  Port=2
  Arbitration : MATLAB Function  TreatAsAtomicUnit=on
  Bus Assignment : BusAssignment  AssignedSignals=ArbitratedActuationReq
  ArbitratedActuationReq : Outport
  ControllerMainBusOut : Outport  Port=2
  wires:
  FeatureReqBus/1 -> Arbitration/1(FunctionFeatures)
  Arbitration/1(ArbitratedReq) -> Bus Assignment/2, ArbitratedActuationReq/1
  ControllerMainBusIn/1 -> Bus Assignment/1
  Bus Assignment/1 -> ControllerMainBusOut/1

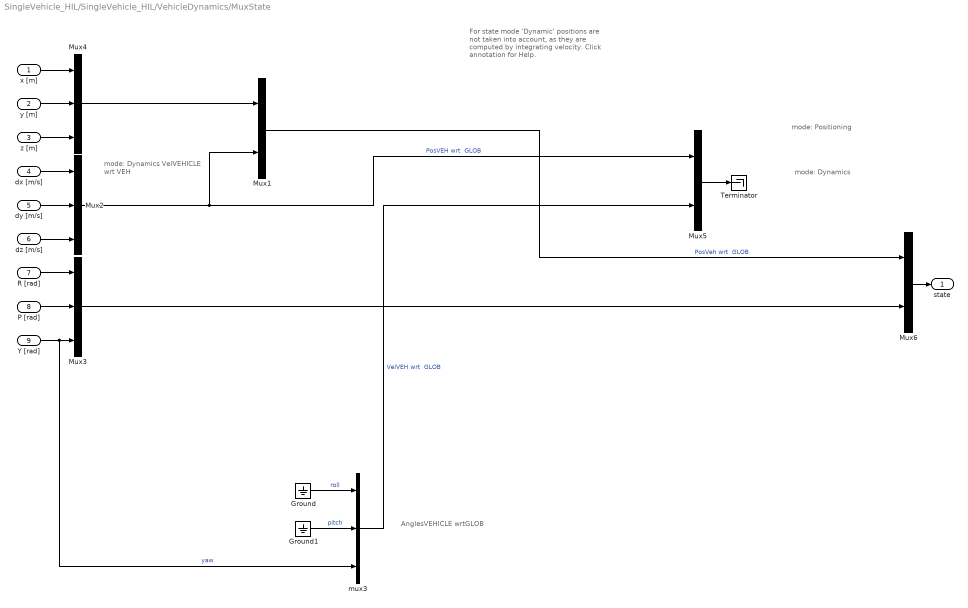
== system SingleVehicle_HIL/SingleVehicle_HIL/VehicleDynamics/MuxState ==
  note: mode: Dynamics
  note: mode: Positioning
  note: mode: Dynamics
      | VelVEHICLE
      | wrt VEH
  note: AnglesVEHICLE
      | wrtGLOB
  note: For state mode 'Dynamic' positions
      | are not taken into account, as they
      | are computed by integrating velocity.
      | Click annotation for Help.
  x [m] : Inport  SampleTime=TimeStep
  y [m] : Inport  Port=2  SampleTime=TimeStep
  z [m] : Inport  Port=3  SampleTime=TimeStep
  dx [m/s] : Inport  Port=4  SampleTime=TimeStep
  dy [m/s] : Inport  Port=5  SampleTime=TimeStep
  dz [m/s] : Inport  Port=6  SampleTime=TimeStep
  R [rad] : Inport  Port=7  SampleTime=TimeStep
  P [rad] : Inport  Port=8  SampleTime=TimeStep
  Y [rad] : Inport  Port=9  SampleTime=TimeStep
  Ground : Ground
  Ground1 : Ground
  Mux1 : Mux  Inputs=[3 3]
  Mux2 : Mux  Inputs=3
  Mux3 : Mux  Inputs=3
  Mux4 : Mux  Inputs=3
  Mux5 : Mux  Inputs=[3 3]
  Mux6 : Mux  Inputs=[6 3]
  Terminator : Terminator
  mux3 : Mux  Inputs=3
  state : Outport
  wires:
  Mux6/1 -> state/1
  Mux4/1 -> Mux1/1
  Mux1/1 -> Mux6/1  "PosVeh wrt  GLOB"
  P [rad]/1 -> Mux3/2
  R [rad]/1 -> Mux3/1
  dz [m/s]/1 -> Mux2/3
  dy [m/s]/1 -> Mux2/2
  dx [m/s]/1 -> Mux2/1
  z [m]/1 -> Mux4/3
  y [m]/1 -> Mux4/2
  x [m]/1 -> Mux4/1
  Ground1/1 -> mux3/2  "pitch"
  Y [rad]/1 -> mux3/3, Mux3/3  "yaw"
  Mux3/1 -> Mux6/2
  mux3/1 -> Mux5/2  "VelVEH wrt  GLOB"
  Ground/1 -> mux3/1  "roll"
  Mux2/1 -> Mux5/1, Mux1/2  "PosVEH wrt  GLOB"
  Mux5/1 -> Terminator/1

== system SingleVehicle_HIL/SingleVehicle_HIL/Controller/Actuation/ActuatorDrivers ==
  ActCmds : Inport
  " Demux " : Demux  Outputs=1
  " SFunction " : S-Function  Tag=Stateflow S-Function $$Clipboard$$ 8  FunctionName=sf_sfun  PortCounts=[1 4]  SFunctionDeploymentMode=off  EnableBusSupport=on
  " Terminator " : Terminator
  accel_cmd : Outport
  decel_cmd : Outport  Port=2
  steering_cmd : Outport  Port=3
  wires:
  ActCmds/1 -> " SFunction "/1
  " SFunction "/2 -> accel_cmd/1  "accel_cmd"
  " SFunction "/3 -> decel_cmd/1  "decel_cmd"
  " SFunction "/4 -> steering_cmd/1  "steering_cmd"
  " Demux "/1 -> " Terminator "/1
  " SFunction "/1 -> " Demux "/1

== system SingleVehicle_HIL/SingleVehicle_HIL/Controller/Actuation/DynamicControls ==
  ActReq : Inport
  Ctl : Inport  Port=2
  ActCmdsPrev : Inport  Port=3
  " Demux " : Demux  Outputs=1
  " SFunction " : S-Function  Tag=Stateflow S-Function $$Clipboard$$ 6  FunctionName=sf_sfun  PortCounts=[3 2]  SFunctionDeploymentMode=off  EnableBusSupport=on
  " Terminator " : Terminator
  ActCmds : Outport
  wires:
  ActReq/1 -> " SFunction "/1
  Ctl/1 -> " SFunction "/2
  ActCmdsPrev/1 -> " SFunction "/3
  " SFunction "/2 -> ActCmds/1  "ActCmds"
  " Demux "/1 -> " Terminator "/1
  " SFunction "/1 -> " Demux "/1

== system SingleVehicle_HIL/SingleVehicle_HIL/Controller/CollectSensorData/IdealSensorsProcess ==
  VehicleState : Inport
  Bus Creator : BusCreator  Inputs=12  OutDataTypeStr=Bus: VehState
  Bus Selector : BusSelector  OutputSignals=x,y,z,theta,phi,psi,u,v,w,dtheta,dphi,dpsi
  IdealSensorsBus : Outport
  wires:
  VehicleState/1 -> Bus Selector/1
  Bus Selector/1 -> Bus Creator/1  "<x>"
  Bus Selector/8 -> Bus Creator/8  "<v>"
  Bus Selector/7 -> Bus Creator/7  "<u>"
  Bus Selector/10 -> Bus Creator/10  "<dtheta>"
  Bus Selector/11 -> Bus Creator/11  "<dphi>"
  Bus Selector/6 -> Bus Creator/6  "<psi>"
  Bus Selector/4 -> Bus Creator/4  "<theta>"
  Bus Selector/9 -> Bus Creator/9  "<w>"
  Bus Selector/2 -> Bus Creator/2  "<y>"
  Bus Selector/5 -> Bus Creator/5  "<phi>"
  Bus Selector/12 -> Bus Creator/12  "<dpsi>"
  Bus Selector/3 -> Bus Creator/3  "<z>"
  Bus Creator/1 -> IdealSensorsBus/1

== system SingleVehicle_HIL/SingleVehicle_HIL/Controller/CollectSensorData/PrescanProcess ==
  PrescanSimData : Inport
  Bus Creator : BusCreator  Inputs=12  OutDataTypeStr=Bus: PrescanSimData
  SELF_Demux : Subsystem  Tag=DemuxSELF  mask(PreScan Demux Block:){}
      settings: DeleteFcn=PreScanBlockDeleteFcn;
      mask Display:
      | port_label('output',1,'x [m]')
      | port_label('output',2,'y [m]')
      | port_label('output',3,'z [m]','texmode','on')
      | port_label('output',4,'Rotx [deg]','texmode','on')
      | port_label('output',5,'Roty [deg]','texmode','on')
      | port_label('output',6,'Rotz [deg]','texmode','on')
      | port_label('output',7,'GPS lat [deg]','texmode','on')
      | port_label('output',8,'GPS long [deg]','texmode','on')
      | port_label('output',9,'GPS alt [m]','texmode','on')
      | port_label('output',10,'Velocity [m/s]')
      | port_label('output',11,'Heading [deg]')
      | port_label('output',12,'Yaw rate [deg/s]')
  PrescanSimDataBus : Outport
  wires:
  SELF_Demux/1(x [m]) -> Bus Creator/1  "x"
  PrescanSimData/1 -> SELF_Demux/1(SELF)
  Bus Creator/1 -> PrescanSimDataBus/1
  SELF_Demux/2(y [m]) -> Bus Creator/2  "y"
  SELF_Demux/3(z [m]) -> Bus Creator/3  "z"
  SELF_Demux/4(rotx [deg]) -> Bus Creator/4  "Rotx"
  SELF_Demux/5(roty [deg]) -> Bus Creator/5  "Roty"
  SELF_Demux/9(GPS alt [m]) -> Bus Creator/9  "GPS_alt"
  SELF_Demux/8(GPS long [deg]) -> Bus Creator/8  "GPS_long"
  SELF_Demux/10(velocity [m/s]) -> Bus Creator/10  "u"
  SELF_Demux/6(rotz [deg]) -> Bus Creator/6  "Rotz"
  SELF_Demux/7(GPS lat [deg]) -> Bus Creator/7  "GPS_lat"
  SELF_Demux/11(heading [deg]) -> Bus Creator/11  "heading"
  SELF_Demux/12(yaw rate [deg/s]) -> Bus Creator/12  "Yaw_rate"

== system SingleVehicle_HIL/SingleVehicle_HIL/Controller/CtlMainBusUnitDelayAndInit/MATLAB Function ==
  u : Inport
  " Demux " : Demux  Outputs=1
  " SFunction " : S-Function  Tag=Stateflow S-Function $$Clipboard$$ 1  FunctionName=sf_sfun  Parameters=veh_struct  PortCounts=[1 2]  SFunctionDeploymentMode=off  EnableBusSupport=on
  " Terminator " : Terminator
  y : Outport
  wires:
  u/1 -> " SFunction "/1
  " SFunction "/2 -> y/1  "y"
  " Demux "/1 -> " Terminator "/1
  " SFunction "/1 -> " Demux "/1

== system SingleVehicle_HIL/SingleVehicle_HIL/Controller/FeaturedFunctions/RHSC ==
  In1 : Inport  PortDimensions=7
  Interpreted MATLAB Function : MATLABFcn  MATLABFcn=RHSC(u(1),u(2),u(3),u(4),u(5),u(6),u(7))
  Out1 : Outport
  wires:
  In1/1 -> Interpreted MATLAB Function/1
  Interpreted MATLAB Function/1 -> Out1/1

== system SingleVehicle_HIL/SingleVehicle_HIL/Controller/FeaturedFunctions/wpFollower ==
  prevWpAction : Inport
  prevSituation : Inport  Port=2
  " Demux " : Demux  Outputs=1
  " SFunction " : S-Function  Tag=Stateflow S-Function $$Clipboard$$ 4  FunctionName=sf_sfun  Parameters=veh_struct  PortCounts=[2 3]  SFunctionDeploymentMode=off  EnableBusSupport=on
  " Terminator " : Terminator
  wpAction : Outport
  newSituation : Outport  Port=2
  wires:
  prevWpAction/1 -> " SFunction "/1
  prevSituation/1 -> " SFunction "/2
  " SFunction "/2 -> wpAction/1  "wpAction"
  " SFunction "/3 -> newSituation/1  "newSituation"
  " Demux "/1 -> " Terminator "/1
  " SFunction "/1 -> " Demux "/1

== system SingleVehicle_HIL/SingleVehicle_HIL/Controller/SituationalAwareness/situationAwareness ==
  prevSituation : Inport
  prescanSimData : Inport  Port=2
  idealSensors : Inport  Port=3
  " Demux " : Demux  Outputs=1
  " SFunction " : S-Function  Tag=Stateflow S-Function $$Clipboard$$ 3  FunctionName=sf_sfun  Parameters=veh_struct  PortCounts=[3 2]  SFunctionDeploymentMode=off  EnableBusSupport=on
  " Terminator " : Terminator
  newSituation : Outport
  wires:
  prevSituation/1 -> " SFunction "/1
  prescanSimData/1 -> " SFunction "/2
  idealSensors/1 -> " SFunction "/3
  " SFunction "/2 -> newSituation/1  "newSituation"
  " Demux "/1 -> " Terminator "/1
  " SFunction "/1 -> " Demux "/1

== system SingleVehicle_HIL/SingleVehicle_HIL/Controller/StrategicArbitration/Arbitration ==
  FunctionFeatures : Inport
  " Demux " : Demux  Outputs=1
  " SFunction " : S-Function  Tag=Stateflow S-Function $$Clipboard$$ 5  FunctionName=sf_sfun  PortCounts=[1 2]  SFunctionDeploymentMode=off  EnableBusSupport=on
  " Terminator " : Terminator
  ArbitratedReq : Outport
  wires:
  FunctionFeatures/1 -> " SFunction "/1
  " SFunction "/2 -> ArbitratedReq/1  "ArbitratedReq"
  " Demux "/1 -> " Terminator "/1
  " SFunction "/1 -> " Demux "/1

== system SingleVehicle_HIL/SingleVehicle_HIL/Subsystem/CollectSensorData/IdealSensorsProcess ==
  VehicleState : Inport
  Bus Creator : BusCreator  Inputs=12  OutDataTypeStr=Bus: VehState
  Bus Selector : BusSelector  OutputSignals=x,y,z,theta,phi,psi,u,v,w,dtheta,dphi,dpsi
  IdealSensorsBus : Outport
  wires:
  VehicleState/1 -> Bus Selector/1
  Bus Selector/1 -> Bus Creator/1  "<x>"
  Bus Selector/8 -> Bus Creator/8  "<v>"
  Bus Selector/7 -> Bus Creator/7  "<u>"
  Bus Selector/10 -> Bus Creator/10  "<dtheta>"
  Bus Selector/11 -> Bus Creator/11  "<dphi>"
  Bus Selector/6 -> Bus Creator/6  "<psi>"
  Bus Selector/4 -> Bus Creator/4  "<theta>"
  Bus Selector/9 -> Bus Creator/9  "<w>"
  Bus Selector/2 -> Bus Creator/2  "<y>"
  Bus Selector/5 -> Bus Creator/5  "<phi>"
  Bus Selector/12 -> Bus Creator/12  "<dpsi>"
  Bus Selector/3 -> Bus Creator/3  "<z>"
  Bus Creator/1 -> IdealSensorsBus/1

== system SingleVehicle_HIL/SingleVehicle_HIL/Subsystem/CollectSensorData/PrescanProcess ==
  PrescanSimData : Inport
  Bus Creator : BusCreator  Inputs=12  OutDataTypeStr=Bus: PrescanSimData
  SELF_Demux : Subsystem  Tag=DemuxSELF  mask(PreScan Demux Block:){}
      settings: DeleteFcn=PreScanBlockDeleteFcn;
      mask Display:
      | port_label('output',1,'x [m]')
      | port_label('output',2,'y [m]')
      | port_label('output',3,'z [m]','texmode','on')
      | port_label('output',4,'Rotx [deg]','texmode','on')
      | port_label('output',5,'Roty [deg]','texmode','on')
      | port_label('output',6,'Rotz [deg]','texmode','on')
      | port_label('output',7,'GPS lat [deg]','texmode','on')
      | port_label('output',8,'GPS long [deg]','texmode','on')
      | port_label('output',9,'GPS alt [m]','texmode','on')
      | port_label('output',10,'Velocity [m/s]')
      | port_label('output',11,'Heading [deg]')
      | port_label('output',12,'Yaw rate [deg/s]')
  PrescanSimDataBus : Outport
  wires:
  SELF_Demux/1(x [m]) -> Bus Creator/1  "x"
  PrescanSimData/1 -> SELF_Demux/1(SELF)
  Bus Creator/1 -> PrescanSimDataBus/1
  SELF_Demux/2(y [m]) -> Bus Creator/2  "y"
  SELF_Demux/3(z [m]) -> Bus Creator/3  "z"
  SELF_Demux/4(rotx [deg]) -> Bus Creator/4  "Rotx"
  SELF_Demux/5(roty [deg]) -> Bus Creator/5  "Roty"
  SELF_Demux/9(GPS alt [m]) -> Bus Creator/9  "GPS_alt"
  SELF_Demux/8(GPS long [deg]) -> Bus Creator/8  "GPS_long"
  SELF_Demux/10(velocity [m/s]) -> Bus Creator/10  "u"
  SELF_Demux/6(rotz [deg]) -> Bus Creator/6  "Rotz"
  SELF_Demux/7(GPS lat [deg]) -> Bus Creator/7  "GPS_lat"
  SELF_Demux/11(heading [deg]) -> Bus Creator/11  "heading"
  SELF_Demux/12(yaw rate [deg/s]) -> Bus Creator/12  "Yaw_rate"

== system SingleVehicle_HIL/SingleVehicle_HIL/Subsystem/FeaturedFunctions/RHSC ==
  In1 : Inport  PortDimensions=7
  Interpreted MATLAB Function : MATLABFcn  MATLABFcn=RHSC(u(1),u(2),u(3),u(4),u(5),u(6),u(7))
  Out1 : Outport
  wires:
  In1/1 -> Interpreted MATLAB Function/1
  Interpreted MATLAB Function/1 -> Out1/1

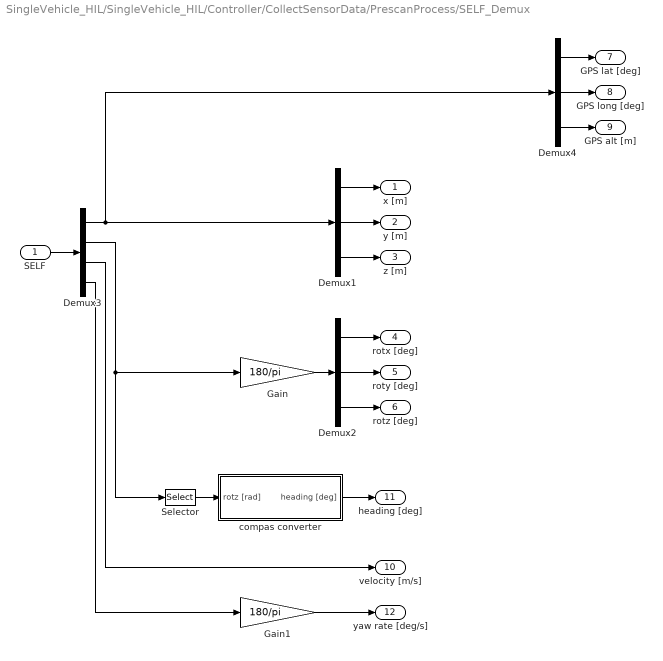
== system SingleVehicle_HIL/SingleVehicle_HIL/Controller/CollectSensorData/PrescanProcess/SELF_Demux ==
  SELF : Inport
  Demux1 : Demux  Outputs=3
  Demux2 : Demux  Outputs=3
  Demux3 : Demux  Outputs=[3 3 1 1]
  Demux4 : Demux  Outputs=3
  Gain : Gain  Gain=180/pi
  Gain1 : Gain  Gain=180/pi
  Selector : Selector  InputPortWidth=3  IndexOptions=Index vector (dialog)  Indices=[3]  OutputSizes=1
  compas converter : Subsystem
  x [m] : Outport
  y [m] : Outport  Port=2
  z [m] : Outport  Port=3
  rotx [deg] : Outport  Port=4
  roty [deg] : Outport  Port=5
  rotz [deg] : Outport  Port=6
  GPS lat [deg] : Outport  Port=7
  GPS long [deg] : Outport  Port=8
  GPS alt [m] : Outport  Port=9
  velocity [m/s] : Outport  Port=10
  heading [deg] : Outport  Port=11
  yaw rate [deg/s] : Outport  Port=12
  wires:
  Demux3/4 -> Gain1/1
  Gain1/1 -> yaw rate [deg/s]/1
  Demux3/3 -> velocity [m/s]/1
  compas converter/1(heading [deg]) -> heading [deg]/1
  Demux3/1 -> Demux4/1, Demux1/1
  Demux4/3 -> GPS alt [m]/1
  Demux4/2 -> GPS long [deg]/1
  Demux4/1 -> GPS lat [deg]/1
  Demux3/2 -> Gain/1, Selector/1
  SELF/1 -> Demux3/1
  Demux2/3 -> rotz [deg]/1
  Demux2/2 -> roty [deg]/1
  Demux2/1 -> rotx [deg]/1
  Demux1/3 -> z [m]/1
  Demux1/2 -> y [m]/1
  Demux1/1 -> x [m]/1
  Gain/1 -> Demux2/1
  Selector/1 -> compas converter/1(rotz [rad])

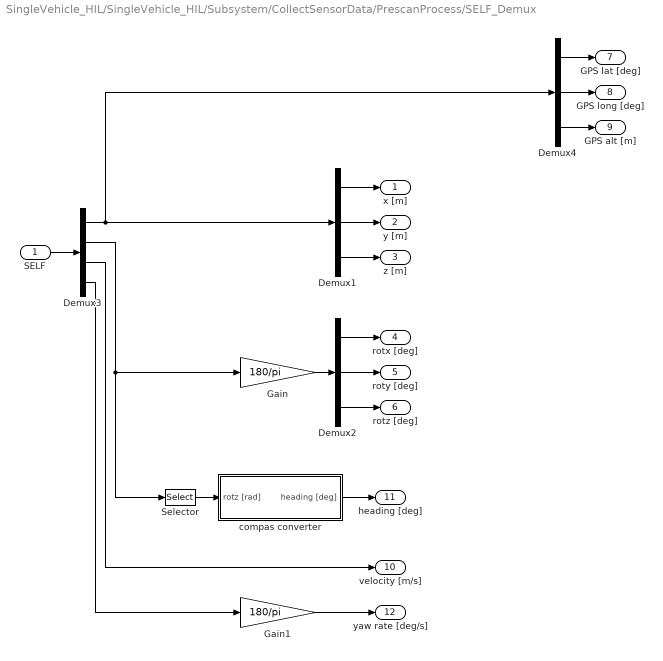
== system SingleVehicle_HIL/SingleVehicle_HIL/Subsystem/CollectSensorData/PrescanProcess/SELF_Demux ==
  SELF : Inport
  Demux1 : Demux  Outputs=3
  Demux2 : Demux  Outputs=3
  Demux3 : Demux  Outputs=[3 3 1 1]
  Demux4 : Demux  Outputs=3
  Gain : Gain  Gain=180/pi
  Gain1 : Gain  Gain=180/pi
  Selector : Selector  InputPortWidth=3  IndexOptions=Index vector (dialog)  Indices=[3]  OutputSizes=1
  compas converter : Subsystem
  x [m] : Outport
  y [m] : Outport  Port=2
  z [m] : Outport  Port=3
  rotx [deg] : Outport  Port=4
  roty [deg] : Outport  Port=5
  rotz [deg] : Outport  Port=6
  GPS lat [deg] : Outport  Port=7
  GPS long [deg] : Outport  Port=8
  GPS alt [m] : Outport  Port=9
  velocity [m/s] : Outport  Port=10
  heading [deg] : Outport  Port=11
  yaw rate [deg/s] : Outport  Port=12
  wires:
  Demux3/4 -> Gain1/1
  Gain1/1 -> yaw rate [deg/s]/1
  Demux3/3 -> velocity [m/s]/1
  compas converter/1(heading [deg]) -> heading [deg]/1
  Demux3/1 -> Demux4/1, Demux1/1
  Demux4/3 -> GPS alt [m]/1
  Demux4/2 -> GPS long [deg]/1
  Demux4/1 -> GPS lat [deg]/1
  Demux3/2 -> Gain/1, Selector/1
  SELF/1 -> Demux3/1
  Demux2/3 -> rotz [deg]/1
  Demux2/2 -> roty [deg]/1
  Demux2/1 -> rotx [deg]/1
  Demux1/3 -> z [m]/1
  Demux1/2 -> y [m]/1
  Demux1/1 -> x [m]/1
  Gain/1 -> Demux2/1
  Selector/1 -> compas converter/1(rotz [rad])

== system SingleVehicle_HIL/SingleVehicle_HIL/Controller/CollectSensorData/PrescanProcess/SELF_Demux/compas converter ==
  rotz [rad] : Inport
  cart2compas : Subsystem
  rad2deg : Gain  Gain=180/pi
  heading [deg] : Outport
  wires:
  cart2compas/1(heading [deg]) -> heading [deg]/1
  rotz [rad]/1 -> rad2deg/1
  rad2deg/1 -> cart2compas/1(Angle [deg])

== system SingleVehicle_HIL/SingleVehicle_HIL/Subsystem/CollectSensorData/PrescanProcess/SELF_Demux/compas converter ==
  rotz [rad] : Inport
  cart2compas : Subsystem
  rad2deg : Gain  Gain=180/pi
  heading [deg] : Outport
  wires:
  cart2compas/1(heading [deg]) -> heading [deg]/1
  rotz [rad]/1 -> rad2deg/1
  rad2deg/1 -> cart2compas/1(Angle [deg])

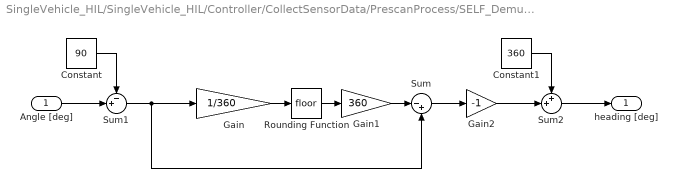
== system SingleVehicle_HIL/SingleVehicle_HIL/Controller/CollectSensorData/PrescanProcess/SELF_Demux/compas converter/cart2compas ==
  Angle [deg] : Inport
  Constant : Constant  Value=90
  Constant1 : Constant  Value=360
  Gain : Gain  Gain=1/360
  Gain1 : Gain  Gain=360
  Gain2 : Gain  Gain=-1
  Rounding Function : Rounding
  Sum : Sum  Inputs=|-+
  Sum1 : Sum  Inputs=-+|
  Sum2 : Sum  Inputs=++|
  heading [deg] : Outport
  wires:
  Sum2/1 -> heading [deg]/1
  Constant1/1 -> Sum2/1
  Gain2/1 -> Sum2/2
  Constant/1 -> Sum1/1
  Sum1/1 -> Sum/2, Gain/1
  Sum/1 -> Gain2/1
  Angle [deg]/1 -> Sum1/2
  Gain1/1 -> Sum/1
  Rounding Function/1 -> Gain1/1
  Gain/1 -> Rounding Function/1

== system SingleVehicle_HIL/SingleVehicle_HIL/Subsystem/CollectSensorData/PrescanProcess/SELF_Demux/compas converter/cart2compas ==
  Angle [deg] : Inport
  Constant : Constant  Value=90
  Constant1 : Constant  Value=360
  Gain : Gain  Gain=1/360
  Gain1 : Gain  Gain=360
  Gain2 : Gain  Gain=-1
  Rounding Function : Rounding
  Sum : Sum  Inputs=|-+
  Sum1 : Sum  Inputs=-+|
  Sum2 : Sum  Inputs=++|
  heading [deg] : Outport
  wires:
  Sum2/1 -> heading [deg]/1
  Constant1/1 -> Sum2/1
  Gain2/1 -> Sum2/2
  Constant/1 -> Sum1/1
  Sum1/1 -> Sum/2, Gain/1
  Sum/1 -> Gain2/1
  Angle [deg]/1 -> Sum1/2
  Gain1/1 -> Sum/1
  Rounding Function/1 -> Gain1/1
  Gain/1 -> Rounding Function/1

== matlab function SingleVehicle_HIL/MATLAB Function ==
  data: u input; y output
function y = fcn(u)
coder.extrinsic('cputime')
persistent t_0
if isempty(t_0)
    t_0 = 0;
    t_0 = cputime;
end
% if not(strcmpi(get_param(test,'SimulationStatus'),'running'))
% t = cputime; 
t = 0;
t = cputime;
y = t - t_0;
% end
end

== matlab function SingleVehicle_HIL/VehStateBusUnitDelayAndInit/MATLAB Function ==
  data: u input; y output Bus: VehState
function y = DelayAndInitVehState(u)
persistent a
y0 = struct;
y0.x = 0;
y0.y = 0;
y0.z = 0;
y0.theta = 0;
y0.phi = 0;
y0.psi = 0;
y0.u = 0;
y0.v = 0;
y0.w = 0;
y0.dtheta = 0;
y0.dphi = 0;
y0.dpsi = 0;

% y0.PWAVehState = struct;
% y0.PWAVehState.Y_PWA = 0;
% y0.PWAVehState.vy_PWA = 0;
% y0.PWAVehState.yaw_angle_PWA = 0;
% y0.PWAVehState.yaw_rate_PWA = 0;

%y0 = VehState_MATLABStruct;
if isempty(a)
    a = 1;
    y = y0;
else
    y = u;
end

== matlab function SingleVehicle_HIL/Subsystem/Actuation/ActuatorDrivers ==
  data: ActCmds input Bus: ActuationCmdBus; accel_cmd output; decel_cmd output; steering_cmd output
function [accel_cmd, decel_cmd, steering_cmd]  = fcn(ActCmds)

accel_cmd = ActCmds.accel_cmd;
decel_cmd = ActCmds.decel_cmd;
steering_cmd = ActCmds.steering_cmd;

end
